simulink library "csu_ptc_vernier_phaseplane_thruster_alloc_lib"  (R2014b)
settings: Solver=ode113  StartTime=0.0  StopTime=10.0  RelTol=1e-3
settings Model: Creator=Jim Kaidy  LastModifiedBy=mstewart

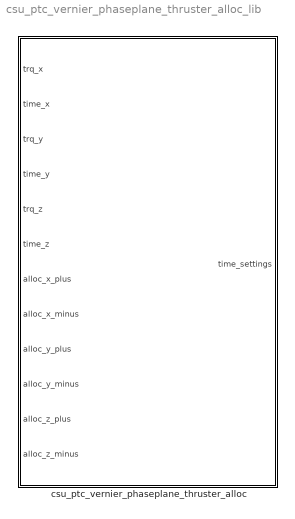
== system csu_ptc_vernier_phaseplane_thruster_alloc_lib ==
  csu_ptc_vernier_phaseplane_thruster_alloc : MATLAB Function  TreatAsAtomicUnit=on

== matlab function csu_ptc_vernier_phaseplane_thruster_alloc_lib/csu_ptc_vernier_phaseplane_thruster_alloc ==
  data: trq_x input; time_x input; trq_y input; time_y input; trq_z input; time_z input; alloc_x_plus input; alloc_x_minus input; alloc_y_plus input; alloc_y_minus input; alloc_z_plus input; alloc_z_minus input; time_settings output
function time_settings  = csu_ptc_vernier_phaseplane_thruster_alloc(trq_x,time_x,trq_y,time_y,trq_z,time_z,alloc_x_plus,alloc_x_minus,alloc_y_plus,alloc_y_minus,alloc_z_plus,alloc_z_minus)
%#codegen

time_settings = uint8(zeros(12,1));

if trq_x == 1
   
    for i = 1:size(alloc_x_plus,1)
        
        time_settings(alloc_x_plus(i)-12,1) = time_x*1000;
        
    end
    
elseif trq_x == -1
    
    for i = 1:size(alloc_x_minus,1)
        
        time_settings(alloc_x_minus(i)-12,1) = time_x*1000;
        
    end    
    
end

if trq_y == 1

    for i = 1:size(alloc_y_plus,1)
 
        time_settings(alloc_y_plus(i)-12,1) = time_y*1000;
        
    end
    
elseif trq_y == -1
    
    for i = 1:size(alloc_y_minus,1)
        
        time_settings(alloc_y_minus(i)-12,1) = time_y*1000;
        
    end    
    
end

if trq_z == 1
   
    for i = 1:size(alloc_z_plus,1)
        
        time_settings(alloc_z_plus(i)-12,1) = time_z*1000;
         
    end
    
elseif trq_z == -1
    
    for i = 1:size(alloc_z_minus,1)
        
        time_settings(alloc_z_minus(i)-12,1) = time_z*1000;
        
    end    
    
end
